simulink model "lab9boostconvdcmmode"  (R2020a)
settings: Solver=VariableStepAuto  StartTime=0.0  StopTime=0.01  RelTol=1e-3
libraries: powerlib x14
settings Model: Creator=Dell  LastModifiedBy=Dell

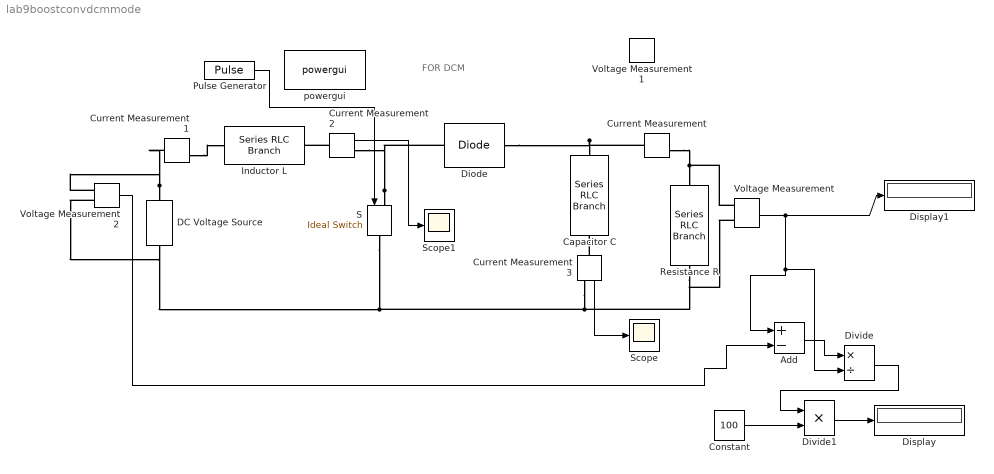
== system lab9boostconvdcmmode ==
  note: FOR DCM
  Add : Sum  Inputs=+-
  Capacitor C : powerlib/Elements/Series RLC Branch  LConnTagsString=__new0  RConnTagsString=__new0  BranchType=C  Resistance=1  Inductance=1e-3  SetiL0=off  InitialCurrent=0  Capacitance=0.00012  Setx0=off  InitialVoltage=0  Measurements=None
  Constant : Constant  Value=100
  Current Measurement{,1..3} (4 alike) : powerlib/Measurements/Current Measurement  PhasorSimulation=off  OutputType=Complex  PSBequivalent=0
  DC Voltage Source : powerlib/Electrical Sources/DC Voltage Source  Amplitude=20  Measurements=None
  "Diode " : powerlib/Power Electronics/Diode  Ron=0.001  Lon=0  Vf=0.8  IC=0  UseSnubber=0  Rs=500  Cs=250e-9  Measurements=off
  Display : Display
  Display1 : Display
  Divide : Product  Inputs=*/
  Divide1 : Product  Inputs=**
  Inductor L : powerlib/Elements/Series RLC Branch  LConnTagsString=__new0  RConnTagsString=__new0  BranchType=L  Resistance=1  Inductance=0.000009  SetiL0=off  InitialCurrent=0  Capacitance=1e-6  Setx0=off  InitialVoltage=0  Measurements=None
  Pulse Generator : DiscretePulseGenerator  PulseType=Time based  Amplitude=10  Period=1/50000  PulseWidth=60
  Resistance R : powerlib/Elements/Series RLC Branch  LConnTagsString=__new0  RConnTagsString=__new0  BranchType=R  Resistance=5  Inductance=1e-3  SetiL0=off  InitialCurrent=0  Capacitance=1e-6  Setx0=off  InitialVoltage=0  Measurements=None
  S : powerlib/Power Electronics/Ideal Switch  Ron=1e-3  Lon=0  IC=0  Rs=1e5  Cs=inf  Measurements=off
  Scope : Scope
  Scope1 : Scope
  Voltage Measurement : powerlib/Measurements/Voltage Measurement  PhasorSimulation=off  OutputType=Complex  PSBequivalent=0
  Voltage Measurement1 : powerlib/Measurements/Voltage Measurement  PhasorSimulation=off  OutputType=Complex  PSBequivalent=0
  Voltage Measurement2 : powerlib/Measurements/Voltage Measurement  PhasorSimulation=off  OutputType=Complex  PSBequivalent=0
  powergui : powerlib/powergui  Priority=1  SimulationMode=Continuous  SampleTime=50e-6  frequency=60  Iterations=50  frequencyindice=0  Pbase=100e6  ErrMax=1e-4  UnitsV=kV  UnitsW=MW  buscounter=0  FunctionMessages=off  echomessages=off  EnableUseOfTLC=off  CurrentSourceSwitches=off  DisableSnubberDevices=off  DisableRonSwitches=off  DisableVfSwitches=off  DisplayEquations=off  AutomaticDiscreteSolvers=off  SolverType=Tustin/Backward Euler (TBE)  Interpol=off  ExternalGateDelay=off  methode=off  Ts=100  x0status=blocks  SPID=on  SwTol=0  HookPort=off  NonlinearTolerance=1e-4  nMaxIteration=100  ContinueOnMaxIteration=off  RestoreLinks=warning  ResistiveCurrentMeasurement=off  Frange=[0:2:500]  Ylog=off  Xlog=on  ShowGrid=off  save=off  variable=ZData  structure=0  ZoomFFT=off  StartTime=0.0  cycles=1  DisplayStyle=1  fundamental=60  FreqAxis=off  MaxFrequency=1000  frequencyindicesteady=1  RmsSteady=1  display=off
  wires:
  Divide1/1 -> Display/1
  Current Measurement2/1 -> Scope1/1
  Current Measurement3/1 -> Scope/1
  Divide/1 -> Divide1/1
  Pulse Generator/1 -> S/1
  Constant/1 -> Divide1/2
  Voltage Measurement/1 -> Divide/2, Add/1, Display1/1
  Add/1 -> Divide/1
  Voltage Measurement2/1 -> Add/2
  connections:
  S/RConn1 -- DC Voltage Source/LConn1 -- Voltage Measurement2/LConn2 -- Current Measurement3/RConn1 -- Voltage Measurement/LConn2 -- Resistance R/RConn1
  S/LConn1 -- "Diode "/LConn1 -- Current Measurement2/RConn1
  Capacitor C/LConn1 -- "Diode "/RConn1 -- Current Measurement/LConn1
  DC Voltage Source/RConn1 -- Current Measurement1/LConn1 -- Voltage Measurement2/LConn1
  Current Measurement/RConn1 -- Voltage Measurement/LConn1 -- Resistance R/LConn1
  Current Measurement2/LConn1 -- Inductor L/RConn1
  Current Measurement3/LConn1 -- Capacitor C/RConn1
  Current Measurement1/RConn1 -- Inductor L/LConn1
